simulink model "DSBt_modulaction"  (R2018a)
settings: Solver=VariableStepAuto  StartTime=0.0  StopTime=50.0  RelTol=1e-3
libraries: dsparch4 x2, commchan3 x1, simulink x1
settings Model: Creator=mengmeng  LastModifiedBy=mengmeng

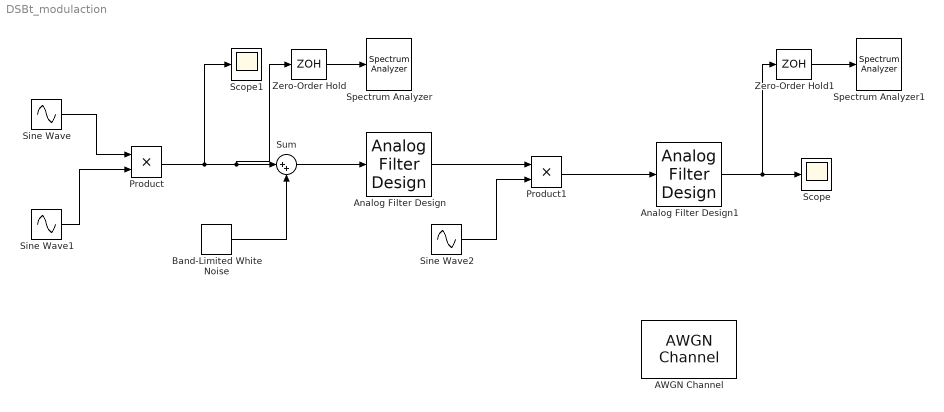
== system DSBt_modulaction ==
  AWGN Channel : commchan3/AWGN Channel  InputProcessing=Columns as channels (frame based)  seed=67  noiseMode="Signal to noise ratio  (Eb/No)"  EbNodB=10  EsNodB=10  SNRdB=10  bitsPerSym=1  Ps=1  Tsym=1  variance=1
  Analog Filter Design : dsparch4/Analog Filter Design  method=Butterworth  filttype=Bandpass  N=8  Wlo=90  Whi=500  Rp=2  Rs=40
  Analog Filter Design1 : dsparch4/Analog Filter Design  method=Butterworth  filttype=Lowpass  N=8  Wlo=10  Whi=80  Rp=2  Rs=40
  Band-Limited White Noise : simulink/Sources/Band-Limited White Noise  Cov=[0]  Ts=0.01  seed=[23341]
  Product : Product
  Product1 : Product
  Scope : Scope
  Scope1 : Scope
  Sine Wave : Sin  Frequency=500  SampleTime=0
  Sine Wave1 : Sin  Frequency=6000  SampleTime=0
  Sine Wave2 : Sin  Frequency=6000  SampleTime=0
  Spectrum Analyzer : SpectrumAnalyzer
  Spectrum Analyzer1 : SpectrumAnalyzer
  Sum : Sum  Inputs=|++
  Zero-Order Hold : ZeroOrderHold  SampleTime=0.01
  Zero-Order Hold1 : ZeroOrderHold  SampleTime=0.01
  wires:
  Sine Wave/1 -> Product/1
  Sine Wave1/1 -> Product/2
  Product/1 -> Scope1/1, Zero-Order Hold/1, Sum/1
  Band-Limited White Noise/1 -> Sum/2
  Sum/1 -> Analog Filter Design/1
  Analog Filter Design/1 -> Product1/1
  Sine Wave2/1 -> Product1/2
  Product1/1 -> Analog Filter Design1/1
  Analog Filter Design1/1 -> Zero-Order Hold1/1, Scope/1
  Zero-Order Hold1/1 -> Spectrum Analyzer1/1
  Zero-Order Hold/1 -> Spectrum Analyzer/1
